simulink model "testRollContSolo"  (R2014a)
settings: Solver=ode45  StartTime=0.0  StopTime=10.0  RelTol=1e-3
undefined symbols (not defined in the file or in its folder): den_tf_cont, motor_den_tf_discrete, motor_num_tf_discrete, num_tf_cont, Whovering
settings Model: Creator=root  LastModifiedBy=root

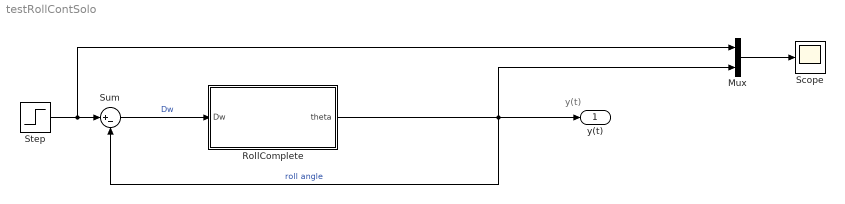
== system testRollContSolo ==
  note: y(t)
  Mux : Mux  Inputs=2
  "RollComplete " : Subsystem
  Scope : Scope
  Step : Step  Time=0  After=40  SampleTime=0
  Sum : Sum  Inputs=|+-
  y(t) : Outport
  wires:
  Step/1 -> Mux/1, Sum/1
  Mux/1 -> Scope/1
  "RollComplete "/1("theta ") -> Mux/2, y(t)/1, Sum/2  "roll angle"
  Sum/1 -> "RollComplete "/1("Dw ")  "Dw"

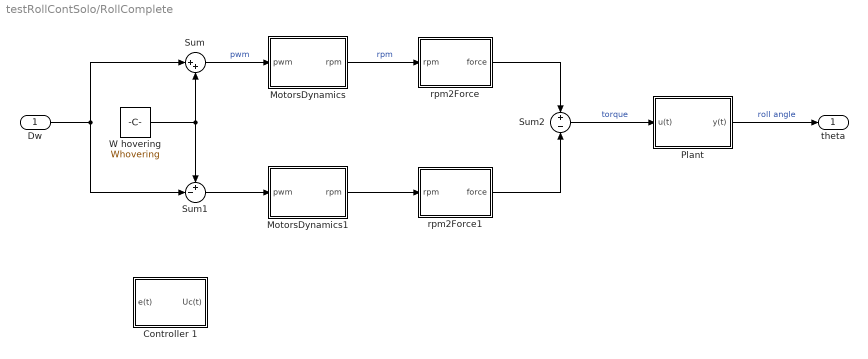
== system testRollContSolo/RollComplete  ==
  "Dw " : Inport
  Controller 1 : Subsystem
  MotorsDynamics : Subsystem
  MotorsDynamics1 : Subsystem
  Plant : Subsystem
  Sum : Sum  Inputs=|++
  Sum1 : Sum  Inputs=+-|
  Sum2 : Sum  Inputs=+|-
  W hovering : Constant  Value=Whovering
  rpm2Force : MATLAB Function  TreatAsAtomicUnit=on
  rpm2Force1 : MATLAB Function  TreatAsAtomicUnit=on
  "theta " : Outport
  wires:
  Plant/1(y(t)) -> "theta "/1  "roll angle"
  "Dw "/1 -> Sum/1, Sum1/2
  Sum2/1 -> Plant/1(u(t))  "torque"
  W hovering/1 -> Sum/2, Sum1/1
  Sum/1 -> MotorsDynamics/1(pwm)  "pwm"
  Sum1/1 -> MotorsDynamics1/1(pwm)
  MotorsDynamics/1(rpm) -> rpm2Force/1(rpm)  "rpm"
  MotorsDynamics1/1(rpm) -> rpm2Force1/1(rpm)
  rpm2Force/1(force) -> Sum2/1
  rpm2Force1/1(force) -> Sum2/2

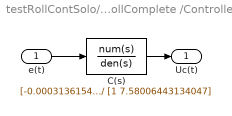
== system testRollContSolo/RollComplete /Controller 1 ==
  e(t) : Inport
  "C(s) " : TransferFcn  Numerator=[-0.00031361544224957 0.0105787614058996]  Denominator=[1 7.58006443134047]
  Uc(t) : Outport
  wires:
  "C(s) "/1 -> Uc(t)/1
  e(t)/1 -> "C(s) "/1

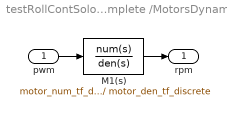
== system testRollContSolo/RollComplete /MotorsDynamics ==
  pwm : Inport
  M1(s) : TransferFcn  Numerator=motor_num_tf_discrete  Denominator=motor_den_tf_discrete  ContinuousStateAttributes='phi'
  rpm : Outport
  wires:
  M1(s)/1 -> rpm/1
  pwm/1 -> M1(s)/1

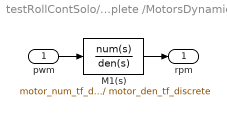
== system testRollContSolo/RollComplete /MotorsDynamics1 ==
  pwm : Inport
  M1(s) : TransferFcn  Numerator=motor_num_tf_discrete  Denominator=motor_den_tf_discrete  ContinuousStateAttributes='phi'
  rpm : Outport
  wires:
  M1(s)/1 -> rpm/1
  pwm/1 -> M1(s)/1

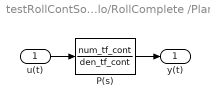
== system testRollContSolo/RollComplete /Plant ==
  u(t) : Inport
  P(s) : TransferFcn  Numerator=num_tf_cont  Denominator=den_tf_cont  ContinuousStateAttributes='phi'
  y(t) : Outport
  wires:
  P(s)/1 -> y(t)/1
  u(t)/1 -> P(s)/1

== matlab function testRollContSolo/RollComplete /rpm2Force1 ==
  data: rpm input; force output
function force = fcn(rpm)
%#codegen

% Computing Thrust force. It is the result of vertical forces acting on all
% blade elements of one propeller
Radius = 0.115 % m
Radius_in = 9 % in
Ct = 0.18
rho = 1.225 % kg/m^3
Aprop = pi*Radius^2

% Convert to RPM
Thrust_newton = Ct*rho*Aprop*(rpm).^2*Radius^2;
Thrust_kg = Thrust_newton/9.81


force = Thrust_newton_3;

== matlab function testRollContSolo/RollComplete /rpm2Force ==
  data: rpm input; force output
function force = fcn(rpm)
%#codegen

% Computing Thrust force. It is the result of vertical forces acting on all
% blade elements of one propeller
Radius = 0.115 % m
Radius_in = 9 % in
Ct = 0.18
rho = 1.225 % kg/m^3
Aprop = pi*Radius^2

% Convert to RPM
Thrust_newton = Ct*rho*Aprop*(rpm).^2*Radius^2;
Thrust_kg = Thrust_newton/9.81


force = Thrust_newton_3;
